simulink model "oClientServer_Model"  (R2024b)
settings: Solver=FixedStepDiscrete  StartTime=0.0  StopTime=10.0  FixedStep=0.05  RelTol=1e-3
settings Model: DataDictionary=DataDictionary.sldd  Creator=fl9990  LastModifiedBy=nabilekhoury
settings OptimizationCC: DefaultParameterBehavior=Inlined  OptimizeBlockIOStorage=off  BufferReuse=off  ReuseModelBlockBuffer=off  GlobalBufferReuse=off  ExpressionFolding=off  EnableMemcpy=off  PassReuseOutputArgsAs=Individual arguments  LocalBlockOutputs=off  ZeroExternalMemoryAtStartup=off  ZeroInternalMemoryAtStartup=off  OptimizeDataStoreBuffers=off  BusAssignmentInplaceUpdate=off  OptimizationLevel=level0  OptimizationCustomize=off  EfficientTunableParamExpr=on
settings DebuggingCC: ParameterTunabilityLossMsg=error
settings ModelReferenceCC: ModelReferenceNumInstancesAllowed=Single
settings SFSimCC: MATLABDynamicMemAlloc=off
settings RTWCC: Description=Embedded Coder  SystemTargetFile=ert.tlc  GenCodeOnly=on  TemplateMakefile=ert_default_tmf  TargetLang=C++
settings CodeAppCC: ForceParamTrailComments=on  IgnoreCustomStorageClasses=off  OperatorAnnotations=on  SimulinkDataObjDesc=on  SFDataObjDesc=on  InsertBlockDesc=on
settings ERTTargetCC: TargetLangStandard=C++17 (ISO)  GenerateSampleERTMain=on  SupportAbsoluteTime=off  CodeInterfacePackaging=C++ class  SupportNonFinite=off  SupportComplex=off  RootIOFormat=Structure reference  ERTCustomFileTemplate=example_file_process.tlc

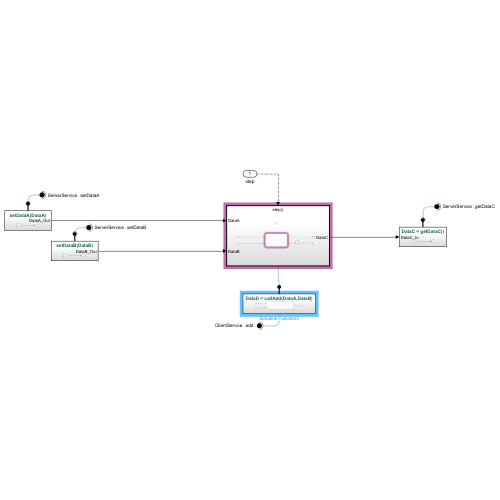
[thumbnail: Simulink's stored preview of the top-level diagram]
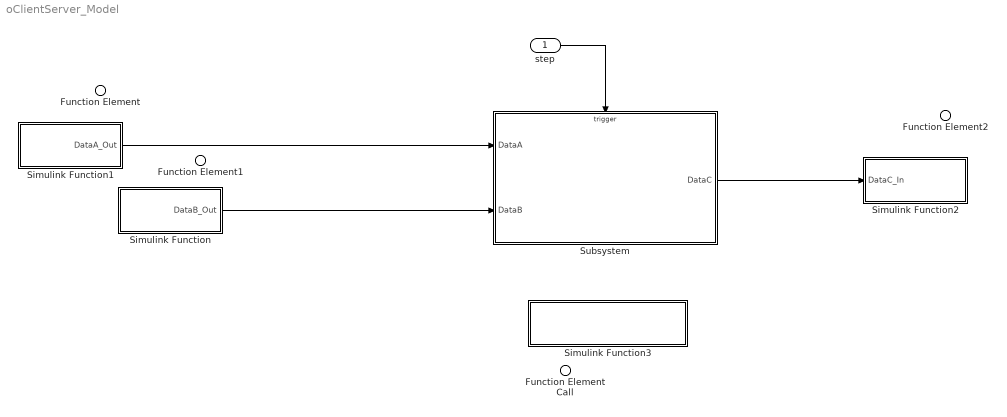
== system oClientServer_Model ==
  step : Inport  OutputFunctionCall=on
  Function Element Call : Inport  Port=2  AllowServiceAccess=on  PortName=ClientService  Element=add
  Simulink Function : Subsystem  TreatAsAtomicUnit=on
  Simulink Function1 : Subsystem  TreatAsAtomicUnit=on
  Simulink Function2 : Subsystem  TreatAsAtomicUnit=on
  Simulink Function3 : Subsystem  TreatAsAtomicUnit=on
  Subsystem : Subsystem
  Function Element2 : Outport  AllowServiceAccess=on  PortName=ServerService  Element=getDataC
  Function Element1 : Outport  AllowServiceAccess=on  PortName=ServerService  Element=setDataB
  Function Element : Outport  AllowServiceAccess=on  PortName=ServerService  Element=setDataA
  wires:
  Simulink Function1/1(DataA_Out) -> Subsystem/1(DataA)
  Simulink Function/1(DataB_Out) -> Subsystem/2(DataB)
  Subsystem/1(DataC) -> Simulink Function2/1(DataC_In)
  step/1 -> Subsystem/Trigger

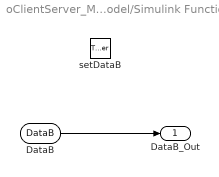
== system oClientServer_Model/Simulink Function ==
  setDataB : TriggerPort  TriggerType=function-call  IsSimulinkFunction=on  FunctionName=setDataB  FunctionVisibility=port  ScopeName=ServerService  VariantControl=(inherit)
  DataB : ArgIn  DisableCoverage=on  ArgumentName=DataB
  DataB_Out : Outport
  wires:
  DataB/1 -> DataB_Out/1

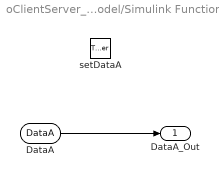
== system oClientServer_Model/Simulink Function1 ==
  setDataA : TriggerPort  TriggerType=function-call  IsSimulinkFunction=on  FunctionName=setDataA  FunctionVisibility=port  ScopeName=ServerService  VariantControl=(inherit)
  DataA : ArgIn  DisableCoverage=on  ArgumentName=DataA
  DataA_Out : Outport
  wires:
  DataA/1 -> DataA_Out/1

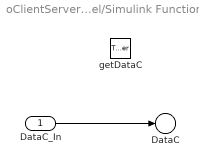
== system oClientServer_Model/Simulink Function2 ==
  DataC_In : Inport
  getDataC : TriggerPort  TriggerType=function-call  IsSimulinkFunction=on  FunctionName=getDataC  FunctionVisibility=port  ScopeName=ServerService  VariantControl=(inherit)
  DataC : ArgOut  ArgumentName=DataC
  wires:
  DataC_In/1 -> DataC/1

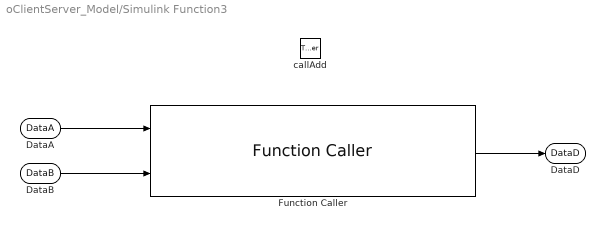
== system oClientServer_Model/Simulink Function3 ==
  callAdd : TriggerPort  TriggerType=function-call  IsSimulinkFunction=on  FunctionName=callAdd  FunctionVisibility=scoped  VariantControl=(inherit)
  Function Caller : FunctionCaller  FunctionPrototype=DataD = ClientService.add(DataA,DataB)  InputArgumentSpecifications=double(1), double(1)  OutputArgumentSpecifications=double(1)
  DataA : ArgIn  DisableCoverage=on  ArgumentName=DataA
  DataB : ArgIn  Port=2  ArgumentName=DataB
  DataD : ArgOut  DisableCoverage=on  ArgumentName=DataD
  wires:
  DataA/1 -> Function Caller/1
  DataB/1 -> Function Caller/2
  Function Caller/1 -> DataD/1

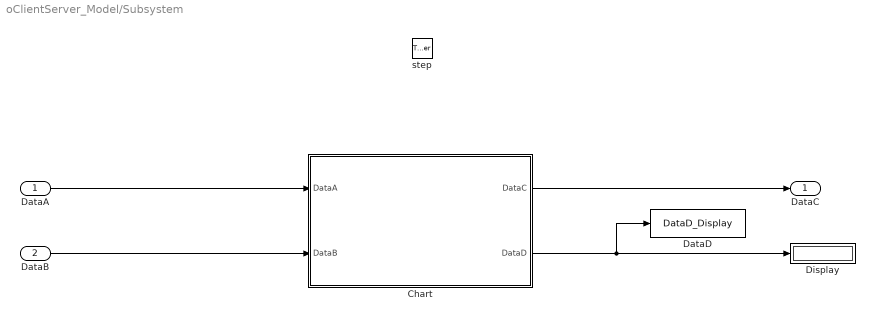
== system oClientServer_Model/Subsystem ==
  DataA : Inport
  DataB : Inport  Port=2
  step : TriggerPort  TriggerType=function-call  VariantControl=(inherit)  PortDimensions=1
  Chart : Stateflow chart  TreatAsAtomicUnit=on
  DataD : DataStoreWrite  DataStoreName=DataD_Display  IndexOptions=Index vector (dialog)  Indices=1  OutputSizes=1
  Display : Display
  DataC : Outport
  wires:
  DataA/1 -> Chart/1(DataA)
  Chart/1(DataC) -> DataC/1
  DataB/1 -> Chart/2(DataB)
  Chart/2(DataD) -> DataD/1, Display/1

== stateflow chart oClientServer_Model/Subsystem/Chart ==
  (default) -> (junction 10)
  (junction 10) -> (junction 11) [order 1] : [DataA > 5]
  (junction 10) -> (junction 12) [order 2] : {
      | DataC = DataA * DataB;
      | }
  (junction 11) -> (junction 13) : {
      | DataC = DataA + DataB;
      | }
  (junction 13) -> (junction 12)
  (junction 12) -> (junction 14) : {
      | DataD = callAdd(DataA, DataB);
      | }
  data: DataA input double size=1; DataB input; DataC output double; DataD output size=1 =0
